simulink model "sfcndemo_mixedmex"  (Simulink 6.0)
settings: Solver=ode5  SolverMode=SingleTasking  StartTime=0.0  StopTime=10.0  FixedStep=.01  RelTol=1e-3
settings Model: Creator=The MathWorks Inc.  LastModifiedBy=batserve  ExtModeTrigMode=oneshot  ExtModeArmWhenConnect=off  ExtModeAutoUpdateStatusClock=off
settings DataIOCC: LimitDataPoints=off
settings OptimizationCC: BooleanDataType=off  InlineInvariantSignals=off
settings DebuggingCC: CheckExecutionContextPreStartOutputMsg=on  CheckExecutionContextRuntimeOutputMsg=on  SolverPrmCheckMsg=none
settings HardwareCC: TargetUnknown=on

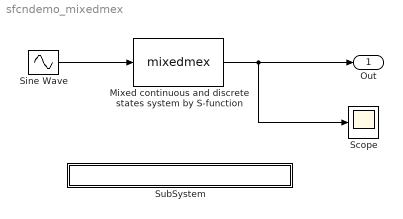
== system sfcndemo_mixedmex ==
  Mixed continuous and discrete states system by S-function : S-Function  FunctionName=mixedmex
      mask Type: S-function: mixedmex
      mask Description: A single-input, single-output system with mixed continuous and discrete states by a S-function.
      mask Display: disp('Single Input\nSingle Output');
  Scope : Scope
      settings: TimeRange=10  YMin=1  YMax=3
  Sine Wave : Sin  SampleTime=0
  SubSystem : Subsystem  PropExecContextAcrossSSBoundary=on
      settings: OpenFcn=edit(fullfile(matlabroot,'simulink','src','mixedmex.c'))
      mask Display: disp('matlabroot\simulink\src\mixedmex.c');
  Out : Outport  InitialOutput=0
  wires:
  Sine Wave/1 -> Mixed continuous and discrete states system by S-function/1
  Mixed continuous and discrete states system by S-function/1 -> Out/1, Scope/1

== system sfcndemo_mixedmex/SubSystem ==
